simulink model "rotation_control_of_drone"  (R2022a)
settings: Solver=VariableStepAuto  StartTime=0.0  StopTime=5  RelTol=1e-3
(part 2 of 2)

== matlab function rotation_control_of_drone/Pole 1 N pole ==
  data: u input; y output; c input
function y = voltage_control(u,c)

y = u*c;

end

== matlab function rotation_control_of_drone/MATLAB Function3 ==
  data: u input; y output; bias input
function y = rotation(u,bias)

if(bias==0)
    y = 1*u;

else
    y = bias*u;

end

end

== matlab function rotation_control_of_drone/MATLAB Function4 ==
  data: u input; y output; bias input
function y = rotation(u,bias)

if(bias==0)
    y = -1*u;

else
    y = bias*u;

end
end

== matlab function rotation_control_of_drone/MATLAB Function5 ==
  data: u input; y output; bias input
function y = rotation(u,bias)

if(bias==0)
    y = -1*u;

else
    y = bias*u;

end

end

== matlab function rotation_control_of_drone/MATLAB Function6 ==
  data: u input; y output; bias input
function y = rotation(u,bias)

if(bias==0)
    y = 1*u;

else
    y = bias*u;

end

end

== matlab function rotation_control_of_drone/Pole 2 N pole ==
  data: u input; y output; c input
function y = voltage_control(u,c)

y = u*c;

end

== matlab function rotation_control_of_drone/Pole 2 S pole ==
  data: u input; y output; c input
function y = voltage_control(u,c)

y = u*c;

end

== matlab function rotation_control_of_drone/Pole 3 N pole ==
  data: u input; y output; c input
function y = voltage_control(u,c)

y = u*c;

end

== matlab function rotation_control_of_drone/Pole 1 S pole ==
  data: u input; y output; c input
function y = voltage_control(u,c)

y = u*c;

end

== matlab function rotation_control_of_drone/Pole 3 S pole ==
  data: u input; y output; c input
function y = voltage_control(u,c)

y = u*c;

end
